simulink model "part2"  (R2021a)
settings: Solver=VariableStepAuto  StartTime=0.0  StopTime=10.0  RelTol=1e-3
values from neighbouring files (symbols this model uses):
  x = input('What is the Temperature in DegX? ')    [part2_run.m]
settings Model: Creator=se7en  LastModifiedBy=se7en

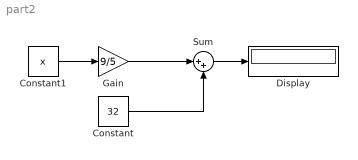
== system part2 ==
  Constant : Constant  Value=32
  Constant1 : Constant  Value=x
  Display : Display
  Gain : Gain  Gain=9/5
  Sum : Sum  Inputs=|++
  wires:
  Gain/1 -> Sum/1
  Constant/1 -> Sum/2
  Sum/1 -> Display/1
  Constant1/1 -> Gain/1
